simulink model "s_pol7"  (Simulink 4.00)
settings: Solver=ode45  SolverMode=SingleTasking  StartTime=0.0  StopTime=200  MaxStep=0.10  RelTol=1e-3  AbsTol=1e-6
values from neighbouring files (symbols this model uses):
  ki = 0.8/ks    [pol4.m]    (also in pol5.m = -Kn(n+1); pol7.m = -Kn(n+1))
settings Model: LastModifiedBy=Administrator  SaveTime=off  SaveOutput=off  LimitDataPoints=off  BlockReductionOpt=off

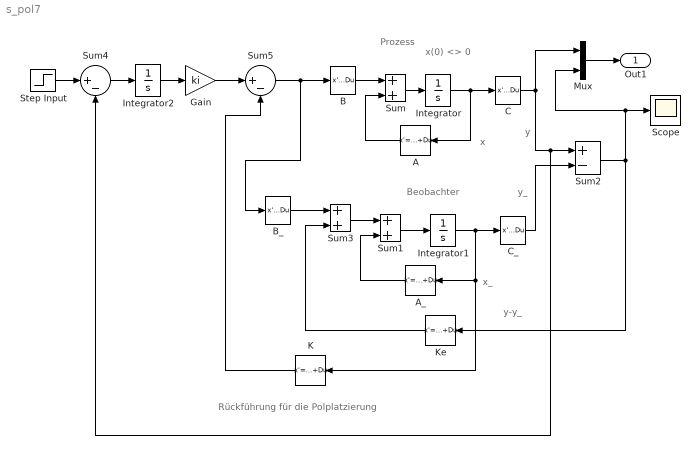
== system s_pol7 ==
  note: x
  note: x_
  note: Beobachter
  note: y
  note: y_
  note: y-y_
  note: x(0) <> 0
  note: Prozess
  note: Rückführung für die
      | Polplatzierung
  A : StateSpace  Orientation=left  A=[]  B=[]  C=[]  D=K  X0=0  Realization=auto  AbsoluteTolerance=auto  mask(Matrix Gain){@1=A}
      mask prompts: @1 "Gain matrix:"
      mask help: Matrix Gain.
      mask init:
      | K = @1;
      mask Help: Multiplies input vector by entered matrix to produce output vector (y=Au).
      mask Display: disp('K')
  A_ : StateSpace  Orientation=left  A=[]  B=[]  C=[]  D=K  X0=0  Realization=auto  AbsoluteTolerance=auto  mask(Matrix Gain){@1=A}
      mask prompts: @1 "Gain matrix:"
      mask help: Matrix Gain.
      mask init:
      | K = @1;
      mask Help: Multiplies input vector by entered matrix to produce output vector (y=Au).
      mask Display: disp('K')
  B : StateSpace  A=[]  B=[]  C=[]  D=K  X0=0  Realization=auto  AbsoluteTolerance=auto  mask(Matrix Gain){@1=B}
      mask prompts: @1 "Gain matrix:"
      mask help: Matrix Gain.
      mask init:
      | K = @1;
      mask Help: Multiplies input vector by entered matrix to produce output vector (y=Au).
      mask Display: disp('K')
  B_ : StateSpace  A=[]  B=[]  C=[]  D=K  X0=0  Realization=auto  AbsoluteTolerance=auto  mask(Matrix Gain){@1=B}
      mask prompts: @1 "Gain matrix:"
      mask help: Matrix Gain.
      mask init:
      | K = @1;
      mask Help: Multiplies input vector by entered matrix to produce output vector (y=Au).
      mask Display: disp('K')
  C : StateSpace  A=[]  B=[]  C=[]  D=K  X0=0  Realization=auto  AbsoluteTolerance=auto  mask(Matrix Gain){@1=C}
      mask prompts: @1 "Gain matrix:"
      mask help: Matrix Gain.
      mask init:
      | K = @1;
      mask Help: Multiplies input vector by entered matrix to produce output vector (y=Au).
      mask Display: disp('K')
  C_ : StateSpace  A=[]  B=[]  C=[]  D=K  X0=0  Realization=auto  AbsoluteTolerance=auto  mask(Matrix Gain){@1=C}
      mask prompts: @1 "Gain matrix:"
      mask help: Matrix Gain.
      mask init:
      | K = @1;
      mask Help: Multiplies input vector by entered matrix to produce output vector (y=Au).
      mask Display: disp('K')
  Gain : Gain  Gain=ki  Multiplication=Element-wise(K.*u)  SaturateOnIntegerOverflow=on
  Integrator : Integrator  ExternalReset=none  InitialConditionSource=internal  InitialCondition=[1 2 1 -2 1 2]  LimitOutput=off  UpperSaturationLimit=inf  LowerSaturationLimit=-inf  ShowSaturationPort=off  ShowStatePort=off  AbsoluteTolerance=auto
  Integrator1 : Integrator  ExternalReset=none  InitialConditionSource=internal  InitialCondition=[0]  LimitOutput=off  UpperSaturationLimit=inf  LowerSaturationLimit=-inf  ShowSaturationPort=off  ShowStatePort=off  AbsoluteTolerance=auto
  Integrator2 : Integrator  ExternalReset=none  InitialConditionSource=internal  InitialCondition=0  LimitOutput=off  UpperSaturationLimit=inf  LowerSaturationLimit=-inf  ShowSaturationPort=off  ShowStatePort=off  AbsoluteTolerance=auto
  K : StateSpace  Orientation=left  A=[]  B=[]  C=[]  D=K  X0=0  Realization=auto  AbsoluteTolerance=auto  mask(Matrix Gain){@1=K}
      mask prompts: @1 "Gain matrix:"
      mask help: Matrix Gain.
      mask init:
      | K = @1;
      mask Help: Multiplies input vector by entered matrix to produce output vector (y=Au).
      mask Display: disp('K')
  Ke : StateSpace  Orientation=left  A=[]  B=[]  C=[]  D=K  X0=0  Realization=auto  AbsoluteTolerance=auto  mask(Matrix Gain){@1=Ke}
      mask prompts: @1 "Gain matrix:"
      mask help: Matrix Gain.
      mask init:
      | K = @1;
      mask Help: Multiplies input vector by entered matrix to produce output vector (y=Au).
      mask Display: disp('K')
  Mux : Mux  Inputs=2
  Scope : Scope
      settings: TickLabels=on  TimeRange=200.000000  YMin=-10.600000  YMax=10.600000  SaveToWorkspace=off  SaveName=ScopeData  DataFormat=Array  LimitDataPoints=on  MaxDataPoints=5000
  Step Input : Step  Time=0  Before=0  After=1  SampleTime=0
  Sum : Sum  Inputs=++  SaturateOnIntegerOverflow=on
  Sum1 : Sum  Inputs=++  SaturateOnIntegerOverflow=on
  Sum2 : Sum  Inputs=+-  SaturateOnIntegerOverflow=on
  Sum3 : Sum  Inputs=++  SaturateOnIntegerOverflow=on
  Sum4 : Sum  Inputs=|+-  SaturateOnIntegerOverflow=on
  Sum5 : Sum  Inputs=|+-  SaturateOnIntegerOverflow=on
  Out1 : Outport  Port=1
  wires:
  Sum2/1 -> Ke/1, Scope/1, Mux/2
  B_/1 -> Sum3/1
  Ke/1 -> Sum3/2
  Sum3/1 -> Sum1/1
  C_/1 -> Sum2/2
  C/1 -> Sum2/1, Sum4/2, Mux/1
  Integrator1/1 -> C_/1, A_/1, K/1
  A_/1 -> Sum1/2
  Sum1/1 -> Integrator1/1
  Integrator/1 -> C/1, A/1
  A/1 -> Sum/2
  Sum/1 -> Integrator/1
  B/1 -> Sum/1
  Step Input/1 -> Sum4/1
  Sum4/1 -> Integrator2/1
  Integrator2/1 -> Gain/1
  Gain/1 -> Sum5/1
  Sum5/1 -> B_/1, B/1
  K/1 -> Sum5/2
  Mux/1 -> Out1/1
